simulink model "PHES_Model_v1"  (R2022a)
settings: Solver=FixedStepAuto  StartTime=0.0  StopTime=inf  FixedStep=1  RelTol=1e-3
values from neighbouring files (symbols this model uses):
  A_1 = 0.006    [Model1_Validation.m]    (also in Run_Model.m = (pi() * penstock_diameter_1^2) / 4)
  A_2 = pi() * R_2^2    [Model1_Validation.m]    (also in Run_Model.m)
  add_loss_factor_gen = pipe_entry_loss + gate_valve_loss_factor + 2*fortyfive_bend_loss + bottom_junction_loss    (= 2.98)    [Model1_Validation.m]    (also in Run_Model.m)
  add_loss_factor_pump = 2*fortyfive_bend_loss + gate_valve_loss_factor    (= 1)    [Model1_Validation.m]    (also in Run_Model.m)
  alpha_1 = i_prop    [Model1_Validation.m]    (also in Run_Model.m = 12)
  beta_1 = 60    [Model1_Validation.m]    (also in Run_Model.m)
  beta_2 = 56    [Model1_Validation.m]    (also in Run_Model.m = 150)
  density = 2500    [Model1_Validation.m]    (also in Run_Model.m = 997)
  fluid_h_inPen = penstock_diameter_1    (= 0.8)    [Model1_Validation.m]    (also in Run_Model.m = 0.6)
  fluid_viscosity = 5.6e-4    (= 0.00056)    [Model1_Validation.m]    (also in Run_Model.m = 0.001)
  g = 9.81    [Model1_Validation.m]    (also in Run_Model.m)
  K_1 = 0    [Model1_Validation.m]    (also in Run_Model.m)
  K_2 = 0    [Model1_Validation.m]    (also in Run_Model.m)
  K_3 = 1    [Model1_Validation.m]    (also in Run_Model.m = 0)
  l_res_alt = 126.3    [Model1_Validation.m]    (also in Run_Model.m)
  l_res_length = 60    [Model1_Validation.m]    (also in Run_Model.m)
  l_res_width = 13    [Model1_Validation.m]    (also in Run_Model.m)
  max_l_res_vol = Set_Vol    (= 2600)    [Model1_Validation.m]    (also in Run_Model.m)
  max_u_res_vol = Set_Vol    (= 2600)    [Model1_Validation.m]    (also in Run_Model.m)
  min_l_res_vol = 20    [Model1_Validation.m]    (also in Run_Model.m)
  min_u_res_vol = 20    [Model1_Validation.m]    (also in Run_Model.m)
  omega = 2*pi()*grid_frq/20    [Model1_Validation.m]    (also in Run_Model.m = 2*pi()*grid_frq)
  penstock_diameter_1 = 0.8    [Model1_Validation.m]    (also in Run_Model.m)
  penstock_length_1 = 380    [Model1_Validation.m]    (also in Run_Model.m)
  penstock_roughness = 1e-5    (= 1e-05)    [Model1_Validation.m]    (also in Run_Model.m; Testing_Cf_iteration.m)
  pump_power_start_1 = 1027000    [Model1_Validation.m]    (also in Run_Model.m)
  R_1 = 0.54    [Model1_Validation.m]    (also in Run_Model.m = 1)
  R_2 = 0.3    [Model1_Validation.m]    (also in Run_Model.m = 0.5)
  turbine_efficiency = 1    [Model1_Validation.m]    (also in Run_Model.m = 0.9)
  u_res_alt = i_height    [Model1_Validation.m]    (also in Run_Model.m = 202.3)
  u_res_length = 60    [Model1_Validation.m]    (also in Run_Model.m)
  u_res_width = 13    [Model1_Validation.m]    (also in Run_Model.m)
  V_init_l_res = 20    [Model1_Validation.m]    (also in Run_Model.m)
  V_init_u_res = Set_Vol    (= 2600)    [Model1_Validation.m]    (also in Run_Model.m)
settings Model: Creator=aasav  LastModifiedBy=aasav
settings SolverCC: InsertRTBMode=Always

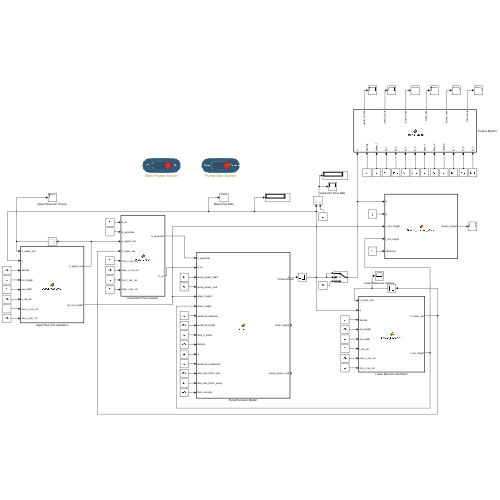
[thumbnail: Simulink's stored preview of the top-level diagram]
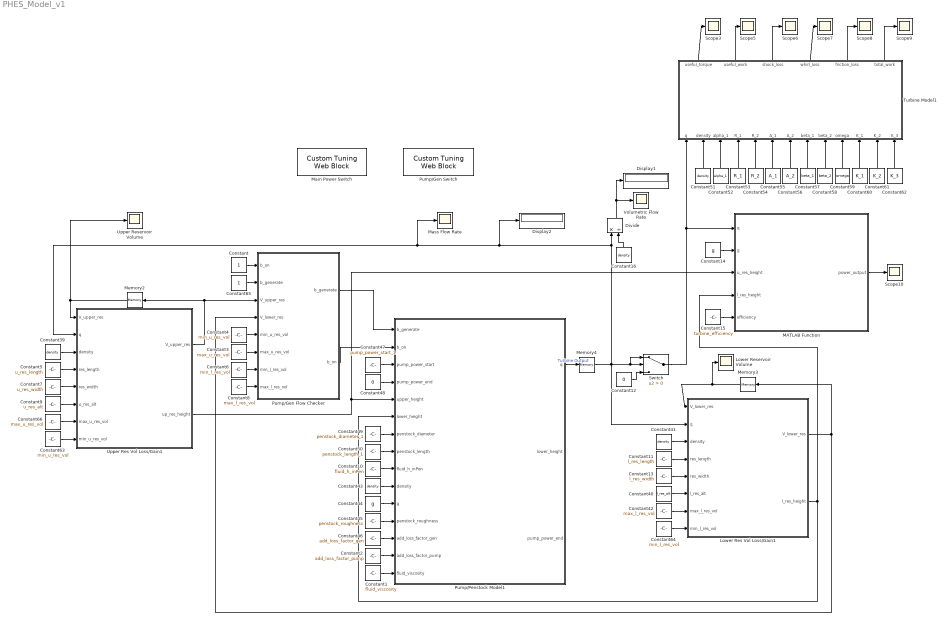
== system PHES_Model_v1 ==
  Constant : Constant
  Constant1 : Constant  Value=fluid_viscosity
  Constant10 : Constant  Value=fluid_h_inPen
  Constant11 : Constant  Value=l_res_length
  Constant12 : Constant  Value=0
  Constant13 : Constant  Value=l_res_width
  Constant14 : Constant  Value=g
  Constant15 : Constant  Value=turbine_efficiency
  Constant{16,39,41,43,51} (5 alike) : Constant  Value=density
  Constant2 : Constant  Value=add_loss_factor_pump
  Constant3 : Constant  Value=max_u_res_vol
  Constant4 : Constant  Value=min_u_res_vol
  Constant40 : Constant  Value=l_res_alt
  Constant42 : Constant  Value=max_l_res_vol
  Constant44 : Constant  Value=g
  Constant45 : Constant  Value=penstock_roughness
  Constant46 : Constant  Value=add_loss_factor_gen
  Constant47 : Constant  Value=pump_power_start_1
  Constant48 : Constant  Value=0
  Constant49 : Constant  Value=penstock_diameter_1
  Constant5 : Constant  Value=u_res_length
  Constant50 : Constant  Value=penstock_length_1
  Constant52 : Constant  Value=alpha_1
  Constant53 : Constant  Value=R_1
  Constant54 : Constant  Value=R_2
  Constant55 : Constant  Value=A_1
  Constant56 : Constant  Value=A_2
  Constant57 : Constant  Value=beta_1
  Constant58 : Constant  Value=beta_2
  Constant59 : Constant  Value=omega
  Constant6 : Constant  Value=min_l_res_vol
  Constant60 : Constant  Value=K_1
  Constant61 : Constant  Value=K_2
  Constant62 : Constant  Value=K_3
  Constant63 : Constant  Value=min_u_res_vol
  Constant64 : Constant  Value=min_l_res_vol
  Constant65 : Constant
  Constant66 : Constant  Value=max_u_res_vol
  Constant7 : Constant  Value=u_res_width
  Constant8 : Constant  Value=max_l_res_vol
  Constant9 : Constant  Value=u_res_alt
  Display1 : Display
  Display2 : Display
  Divide : Product  Inputs=*/
  Lower Res Vol Loss/Gain1 : MATLAB Function  TreatAsAtomicUnit=on
  Lower Reservoir Volume : Scope
  MATLAB Function : MATLAB Function  TreatAsAtomicUnit=on
  Main Power Switch : CustomTuningWebBlock  LabelPosition=Hide  ShowInitialText=on  Configuration="{\"components\":[{\"name\":\"CustomSwitchStateComponent\",\"settings\":{\"position\":[0,0,1,1],\"states\":[{\"HitRegion\":{\"position\":[0,0,0.5,1]},\"Image\":{\"position\":[0,0,1,1],\"size\":[1,1],\"src\":\"data:image\\/svg+xml;base64,PD94bWwgdmVyc2lvbj0iMS4wIiBlbmNvZGluZz0idXRmLTgiPz4NCjwhLS0gR2VuZXJhdG9yOiBBZG9iZSBJbGx1c3RyYXRvciAyNS4yLjEsIFNWRyBFeHBvcnQgUGx1Zy1JbiAuIFNWRyBWZXJzaW9uOiA2LjAwIEJ1aWxkIDApICAtLT4NCjxzdmcgdmVyc2lvbj0iMS4xIiB4bWxucz0iaHR0cDovL3d3dy53My5vcmcvMjAwMC9zdmciIHhtbG5zOnhsaW5rPSJodHRwOi8vd3d3LnczLm9yZy8xOTk5L3hsaW5rIiB4PSIwcHgiIHk9IjBweCINCgkgdmlld0JveD0iMCAwIDc2IDI5IiBzdHlsZT0iZW5hYmxlLWJhY2tncm91bmQ6bmV3 ...(+5404 chars)\",\"srcOrientation\":\"Right\"},\"Label\":{\"color\":[0.9882352941176471,0.9882352941176471,0.7725490196078432],\"icon\":{\"size\":[0,0],\"src\":[],\"srcOrientation\":\"Right\"},\"iconPlacement\":\"left\",\"opacity\":1,\"position\":[0.5,0.14],\"show\":true,\"text\":{\"content\":\"Off\",\"font\":\"Helvetica\",\"fontSize\":14}},\"Value\":0},{\"HitRegion\":{\"position\":[0,0.5,0.5,1]},\"Image\":{\"position\":[0,0,1,1],\"size\":[1,1],\"src\":\"data:image\\/svg+xml;base64,PD94bWwgdmVyc2lvbj0iMS4wIiBlbmNvZGluZz0idXRmLTgiPz4NCjwhLS0gR2VuZXJhdG9yOiBBZG9iZSBJbGx1c3RyYXRvciAyNS4yLjEsIFNWRyBFeHBvcnQgUGx1Zy1JbiAuIFNWRyBWZXJzaW9uOiA2LjAwIEJ1aWxkIDApICAtLT4NCjxzdmcgdmVyc2lvbj0iMS4xIiB4bWxucz0iaHR0cDovL3d3dy53My5vcmcvMjAwMC9zdmciIHhtbG5zOnhsaW5rPSJodHRwOi8vd3d3LnczLm9yZy8xOTk5L3hsaW5rIiB4PSIwcHgiIHk9IjBweCINCgkgdmlld0JveD0iMCAwIDc2IDI5IiBzdHlsZT0iZW5hYmxlLWJhY2tncm91bmQ6bmV3 ...(+5404 chars)\",\"srcOrientation\":\"Right\"},\"Label\":{\"color\":[0.9882352941176471,0.9882352941176471,0.7725490196078432],\"icon\":{\"size\":[0,0],\"src\":[],\"srcOrientation\":\"Right\"},\"iconPlacement\":\"left\",\"opacity\":1,\"position\":[0.5,0.86],\"show\":true,\"text\":{\"content\":\"On\",\"font\":\"Helvetica\",\"fontSize\":14}},\"Value\":1}]}},{\"name\":\"BackgroundImageComponent\",\"settings\":{\"image\":{\"size\":[140,55],\"src\":\"default\",\"srcOrientation\":\"Right\"},\"position\":[0,0,1,1],\"scaleMode\":\"0\"}},{\"name\":\"ForegroundImageComponent\",\"settings\":{\"image\":{\"size\":[0,0],\"src\":\"default\",\"srcOrientation\":[]},\"isForeground\":1,\"position\":[0,0,1,1],\"scaleMode\":\"0\"}}],\"settings\":{\"BindingType\":\"param\",\"backgroundColor\":[0,0,255,\"1\"],\"backgroundOffset\":0.14,\"fixedAspectRatio\":\"on\",\"foregroundColor\":[234,234,234],\"showBackgroundColor\":false,\"variant\":\"slider\"},\"type\":\"Switch\"}"
  Mass Flow Rate : Scope
  Memory2 : Memory  InitialCondition=V_init_u_res
  Memory3 : Memory  InitialCondition=V_init_l_res
  Memory4 : Memory  InheritSampleTime=on
  Pump/Gen Flow Checker : MATLAB Function  TreatAsAtomicUnit=on
  Pump/Gen Switch : CustomTuningWebBlock  LabelPosition=Hide  ShowInitialText=on  Configuration="{\"components\":[{\"name\":\"CustomSwitchStateComponent\",\"settings\":{\"position\":[0,0,1,1],\"states\":[{\"HitRegion\":{\"position\":[0,0,0.5,1]},\"Image\":{\"position\":[0,0,1,1],\"size\":[1,1],\"src\":\"data:image\\/svg+xml;base64,PD94bWwgdmVyc2lvbj0iMS4wIiBlbmNvZGluZz0idXRmLTgiPz4NCjwhLS0gR2VuZXJhdG9yOiBBZG9iZSBJbGx1c3RyYXRvciAyNS4yLjEsIFNWRyBFeHBvcnQgUGx1Zy1JbiAuIFNWRyBWZXJzaW9uOiA2LjAwIEJ1aWxkIDApICAtLT4NCjxzdmcgdmVyc2lvbj0iMS4xIiB4bWxucz0iaHR0cDovL3d3dy53My5vcmcvMjAwMC9zdmciIHhtbG5zOnhsaW5rPSJodHRwOi8vd3d3LnczLm9yZy8xOTk5L3hsaW5rIiB4PSIwcHgiIHk9IjBweCINCgkgdmlld0JveD0iMCAwIDc2IDI5IiBzdHlsZT0iZW5hYmxlLWJhY2tncm91bmQ6bmV3 ...(+5404 chars)\",\"srcOrientation\":\"Right\"},\"Label\":{\"color\":[0.9882352941176471,0.9882352941176471,0.7725490196078432],\"icon\":{\"size\":[0,0],\"src\":[],\"srcOrientation\":\"Right\"},\"iconPlacement\":\"left\",\"opacity\":1,\"position\":[0.5,0.14],\"show\":true,\"text\":{\"content\":\"Pump\",\"font\":\"Helvetica\",\"fontSize\":14}},\"Value\":0},{\"HitRegion\":{\"position\":[0,0.5,0.5,1]},\"Image\":{\"position\":[0,0,1,1],\"size\":[1,1],\"src\":\"data:image\\/svg+xml;base64,PD94bWwgdmVyc2lvbj0iMS4wIiBlbmNvZGluZz0idXRmLTgiPz4NCjwhLS0gR2VuZXJhdG9yOiBBZG9iZSBJbGx1c3RyYXRvciAyNS4yLjEsIFNWRyBFeHBvcnQgUGx1Zy1JbiAuIFNWRyBWZXJzaW9uOiA2LjAwIEJ1aWxkIDApICAtLT4NCjxzdmcgdmVyc2lvbj0iMS4xIiB4bWxucz0iaHR0cDovL3d3dy53My5vcmcvMjAwMC9zdmciIHhtbG5zOnhsaW5rPSJodHRwOi8vd3d3LnczLm9yZy8xOTk5L3hsaW5rIiB4PSIwcHgiIHk9IjBweCINCgkgdmlld0JveD0iMCAwIDc2IDI5IiBzdHlsZT0iZW5hYmxlLWJhY2tncm91bmQ6bmV3 ...(+5404 chars)\",\"srcOrientation\":\"Right\"},\"Label\":{\"color\":[0.9882352941176471,0.9882352941176471,0.7725490196078432],\"icon\":{\"size\":[0,0],\"src\":[],\"srcOrientation\":\"Right\"},\"iconPlacement\":\"left\",\"opacity\":1,\"position\":[0.5,0.86],\"show\":true,\"text\":{\"content\":\"Generate\",\"font\":\"Helvetica\",\"fontSize\":14}},\"Value\":1}]}},{\"name\":\"BackgroundImageComponent\",\"settings\":{\"image\":{\"size\":[140,55],\"src\":\"default\",\"srcOrientation\":\"Right\"},\"position\":[0,0,1,1],\"scaleMode\":\"0\"}},{\"name\":\"ForegroundImageComponent\",\"settings\":{\"image\":{\"size\":[0,0],\"src\":\"default\",\"srcOrientation\":[]},\"isForeground\":1,\"position\":[0,0,1,1],\"scaleMode\":\"0\"}}],\"settings\":{\"BindingType\":\"param\",\"backgroundColor\":[0,0,255,\"1\"],\"backgroundOffset\":0.14,\"fixedAspectRatio\":\"on\",\"foregroundColor\":[234,234,234],\"showBackgroundColor\":false,\"variant\":\"slider\"},\"type\":\"Switch\"}"
  Pump/Penstock Model1 : MATLAB Function  TreatAsAtomicUnit=on
  Scope{3,5..10} (7 alike) : Scope
  Switch : Switch  Criteria=u2 > Threshold  SaturateOnIntegerOverflow=off  InputSameDT=off
  Turbine Model1 : MATLAB Function  TreatAsAtomicUnit=on
  Upper Res Vol Loss/Gain1 : MATLAB Function  TreatAsAtomicUnit=on
  Upper Reservoir Volume : Scope
  Volumetric Flow Rate : Scope
  wires:
  Constant5/1 -> Upper Res Vol Loss/Gain1/4(res_length)
  Constant7/1 -> Upper Res Vol Loss/Gain1/5(res_width)
  Constant9/1 -> Upper Res Vol Loss/Gain1/6(u_res_alt)
  Constant39/1 -> Upper Res Vol Loss/Gain1/3(density)
  Upper Res Vol Loss/Gain1/1(V_upper_res) -> Memory2/1, Pump/Gen Flow Checker/3(V_upper_res)
  Memory2/1 -> Upper Reservoir Volume/1, Upper Res Vol Loss/Gain1/1("V_upper_res ")
  Memory3/1 -> Lower Reservoir Volume/1, Lower Res Vol Loss/Gain1/1("V_lower_res ")
  Constant42/1 -> Lower Res Vol Loss/Gain1/7(max_l_res_vol)
  Constant11/1 -> Lower Res Vol Loss/Gain1/4(res_length)
  Constant41/1 -> Lower Res Vol Loss/Gain1/3(density)
  Constant40/1 -> Lower Res Vol Loss/Gain1/6(l_res_alt)
  Lower Res Vol Loss/Gain1/1(V_lower_res) -> Memory3/1, Pump/Gen Flow Checker/4(V_lower_res)
  Constant13/1 -> Lower Res Vol Loss/Gain1/5(res_width)
  Constant47/1 -> Pump/Penstock Model1/3(pump_power_start)
  Constant48/1 -> Pump/Penstock Model1/4("pump_power_end ")
  Constant49/1 -> Pump/Penstock Model1/7(penstock_diameter)
  Constant50/1 -> Pump/Penstock Model1/8(penstock_length)
  Constant43/1 -> Pump/Penstock Model1/10(density)
  Constant44/1 -> Pump/Penstock Model1/11(g)
  Constant45/1 -> Pump/Penstock Model1/12(penstock_roughness)
  Constant46/1 -> Pump/Penstock Model1/13(add_loss_factor_gen)
  Constant51/1 -> Turbine Model1/2(density)
  Constant62/1 -> Turbine Model1/13(K_3)
  Constant59/1 -> Turbine Model1/10(omega)
  Constant57/1 -> Turbine Model1/8(beta_1)
  Constant61/1 -> Turbine Model1/12(K_2)
  Constant58/1 -> Turbine Model1/9(beta_2)
  Constant54/1 -> Turbine Model1/5(R_2)
  Constant53/1 -> Turbine Model1/4(R_1)
  Constant55/1 -> Turbine Model1/6(A_1)
  Constant52/1 -> Turbine Model1/3(alpha_1)
  Pump/Penstock Model1/1(q) -> Memory4/1  "Turbine Output"
  Constant60/1 -> Turbine Model1/11(K_1)
  Constant56/1 -> Turbine Model1/7(A_2)
  Pump/Gen Flow Checker/1(b_generate) -> Pump/Penstock Model1/1(b_generate)
  Upper Res Vol Loss/Gain1/2(up_res_height) -> Pump/Penstock Model1/5(upper_height), MATLAB Function/3(u_res_height)
  Lower Res Vol Loss/Gain1/2(l_res_height) -> Pump/Penstock Model1/6("lower_height "), MATLAB Function/4(l_res_height)
  Pump/Gen Flow Checker/2(b_on) -> Pump/Penstock Model1/2(b_on)
  Memory4/1 -> Switch/1, Switch/2, Upper Res Vol Loss/Gain1/2(q), Mass Flow Rate/1, Display2/1, Divide/1, Lower Res Vol Loss/Gain1/2(q)
  Constant63/1 -> Upper Res Vol Loss/Gain1/8(min_u_res_vol)
  Constant64/1 -> Lower Res Vol Loss/Gain1/8(min_l_res_vol)
  Constant66/1 -> Upper Res Vol Loss/Gain1/7(max_u_res_vol)
  Constant1/1 -> Pump/Penstock Model1/15(fluid_viscosity)
  Constant2/1 -> Pump/Penstock Model1/14(add_loss_factor_pump)
  Constant/1 -> Pump/Gen Flow Checker/1("b_on ")
  Constant65/1 -> Pump/Gen Flow Checker/2("b_generate ")
  Constant3/1 -> Pump/Gen Flow Checker/6(max_u_res_vol)
  Constant4/1 -> Pump/Gen Flow Checker/5(min_u_res_vol)
  Constant6/1 -> Pump/Gen Flow Checker/7(min_l_res_vol)
  Constant8/1 -> Pump/Gen Flow Checker/8(max_l_res_vol)
  Switch/1 -> Turbine Model1/1(q), MATLAB Function/1(q)
  Turbine Model1/1(useful_torque) -> Scope3/1
  Turbine Model1/2(useful_work) -> Scope5/1
  Turbine Model1/3(shock_loss) -> Scope6/1
  Turbine Model1/4(whirl_loss) -> Scope7/1
  Turbine Model1/5(friction_loss) -> Scope8/1
  Turbine Model1/6(total_work) -> Scope9/1
  Constant12/1 -> Switch/3
  Constant14/1 -> MATLAB Function/2(g)
  Constant15/1 -> MATLAB Function/5(efficiency)
  MATLAB Function/1(power_output) -> Scope10/1
  Constant10/1 -> Pump/Penstock Model1/9(fluid_h_inPen)
  Constant16/1 -> Divide/2
  Divide/1 -> Display1/1, Volumetric Flow Rate/1

== matlab function PHES_Model_v1/Turbine Model1 ==
  data: q input; useful_torque output; density input; alpha_1 input; R_1 input; R_2 input; A_1 input; A_2 input; beta_1 input; beta_2 input; omega input; K_1 input; K_2 input; useful_work output; shock_loss output; whirl_loss output; friction_loss output; total_work output; K_3 input
function [useful_torque, useful_work, shock_loss, whirl_loss, friction_loss, total_work] = Turbine_Model(q, density, alpha_1, R_1, R_2, A_1, A_2, beta_1, beta_2, omega, K_1, K_2, K_3)

    [useful_torque, useful_work, shock_loss, whirl_loss, friction_loss, total_work] = turbine_eqn(q, density, alpha_1, R_1, R_2, A_1, A_2, beta_1, beta_2, omega, K_1, K_2, K_3);

== matlab function PHES_Model_v1/Upper Res Vol Loss//Gain1 ==
  data: V_upper_res output; V_upper_res input; q input; density input; res_length input; res_width input; up_res_height output; u_res_alt input; max_u_res_vol input; min_u_res_vol input
function [V_upper_res, up_res_height] = Upper_Reservoir(V_upper_res, q, density, res_length, res_width, u_res_alt, max_u_res_vol, min_u_res_vol)

    [V_upper_res, up_res_height] = fcn_vol_upper(V_upper_res, q, density, res_length, res_width, u_res_alt, max_u_res_vol, min_u_res_vol);

== matlab function PHES_Model_v1/Pump//Gen Flow Checker ==
  data: b_generate output; b_on input; b_generate input; b_on output; V_upper_res input; V_lower_res input; min_u_res_vol input; max_u_res_vol input; min_l_res_vol input; max_l_res_vol input
function [b_generate, b_on] = Flow_Check(b_on, b_generate, V_upper_res, V_lower_res, min_u_res_vol, max_u_res_vol, min_l_res_vol, max_l_res_vol)
    % Function that dictates whether there is any flow available 
    
    if b_on
        if b_generate
            if ~(V_upper_res > min_u_res_vol && V_lower_res < max_l_res_vol)
                b_on = 0;
            end
        else
            if ~(V_upper_res < max_u_res_vol && V_lower_res > min_l_res_vol)
                b_on = 0;
            end
        end
    end

== matlab function PHES_Model_v1/MATLAB Function ==
  data: q input; power_output output; g input; u_res_height input; l_res_height input; efficiency input
function power_output = Simple_Turbine_Model(q, g, u_res_height, l_res_height, efficiency)

    power_output = simple_turbine_eqn(q, g, u_res_height, l_res_height, efficiency);

== matlab function PHES_Model_v1/Pump//Penstock Model1 ==
  data: b_generate input; b_on input; pump_power_start input; q output; lower_height output; pump_power_end input; upper_height input; lower_height input; penstock_diameter input; penstock_length input; fluid_h_inPen input; density input; g input; penstock_roughness input; pump_power_end output; add_loss_factor_gen input; add_loss_factor_pump input; fluid_viscosity input
function [q, lower_height, pump_power_end] = Penstock(b_generate, b_on, pump_power_start, pump_power_end, upper_height, lower_height, penstock_diameter, penstock_length, fluid_h_inPen, density, g, penstock_roughness, add_loss_factor_gen, add_loss_factor_pump, fluid_viscosity)

    if b_on
        if b_generate
            % Set potential gain to positive
            potential_gain = density * g * (upper_height - lower_height);
    
            % No pumping occurs
            pump_pressure_gain = 0;

            % Set the valve loss factor
            add_loss_factor = add_loss_factor_gen;
        else
            % Flow from lower to upper so negative potential gain
            potential_gain = density * g * (lower_height - upper_height);
    
            % Pumping pressure is induced
            pump_pressure_gain = pump_power_start-pump_power_end;

            % Set the valve loss factor
            add_loss_factor = add_loss_factor_pump;
        end

        segment_theta = 2*acos(1-((2*fluid_h_inPen)/penstock_diameter));

        penstock_diameter = sqrt((penstock_diameter^2 * (segment_theta - sin(segment_theta)))/(2*pi()));

        pressure_gain = pump_pressure_gain + potential_gain;

        q = fcn_penstock_steadystate(pressure_gain, penstock_diameter, penstock_length, density, penstock_roughness, add_loss_factor, fluid_viscosity);
    
        if ~b_generate
            q = -q;
        end
    else
        q = 0;
    end

== matlab function PHES_Model_v1/Lower Res Vol Loss//Gain1 ==
  data: V_lower_res input; V_lower_res output; q input; density input; res_length input; res_width input; l_res_height output; l_res_alt input; max_l_res_vol input; min_l_res_vol input
function [V_lower_res, l_res_height] = Lower_Reservoir(V_lower_res, q, density, res_length, res_width, l_res_alt, max_l_res_vol, min_l_res_vol)

    [V_lower_res, l_res_height] = fcn_vol_lower(V_lower_res, q, density, res_length, res_width, l_res_alt, max_l_res_vol, min_l_res_vol);
